simulink model "luenberg_observers"  (R2024b)
settings: Solver=VariableStepAuto  StartTime=0.0  StopTime=400  RelTol=1e-3
values from neighbouring files (symbols this model uses):
  An = double(subs(Af,{M,m1,m2,l1,l2,g},{1000,100,100,20,10,9.81}))    [PartD_LQRController.m]    (also in PartF_luenberger_observers.m; PartG_LQG_controller.m)
  Bn = double(subs(Bf,{M,m1,m2,l1,l2,g},{1000,100,100,20,10,9.81}))    [PartD_LQRController.m]    (also in PartF_luenberger_observers.m; PartG_LQG_controller.m)
  C1 = [ 0 0 0 0 0 0 ... (first row only)    [PartE_observbliltiy_check.m]    (also in PartF_luenberger_observers.m)
  C3 = [ 0 0 0 0 0 0 ... (first row only)    [PartE_observbliltiy_check.m]    (also in PartF_luenberger_observers.m)
  C4 = [ 0 0 0 0 0 0 ... (first row only)    [PartE_observbliltiy_check.m]    (also in PartF_luenberger_observers.m)
  D = [0;0;0;0;0;0]    [PartB_linearization.m]    (also in PartC_contollability_condition.m; PartD_LQRController.m; PartE_observbliltiy_check.m; PartF_luenberger_observers.m)
  x0 = [0;0;0;0;0.1;-0.1]    [PartB_linearization.m]    (also in PartC_contollability_condition.m = [0;0;0;0;0;0]; PartD_LQRController.m = [0;0;0;5;0;0]; PartE_observbliltiy_check.m = [0;0;0;0;0;0]; PartF_luenberger_observers.m = [0;0;0;0;0;0])
libraries: eeLuenbergerObserver x6

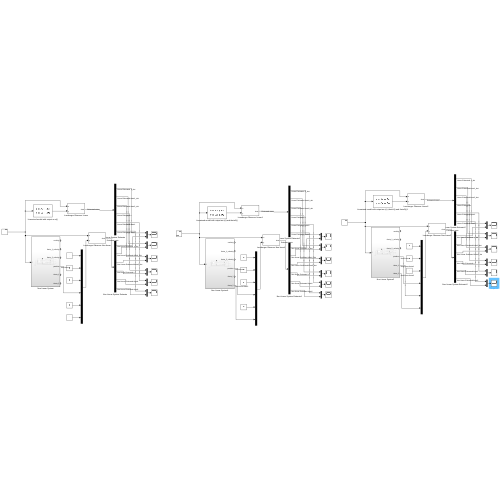
[thumbnail: Simulink's stored preview of the top-level diagram]
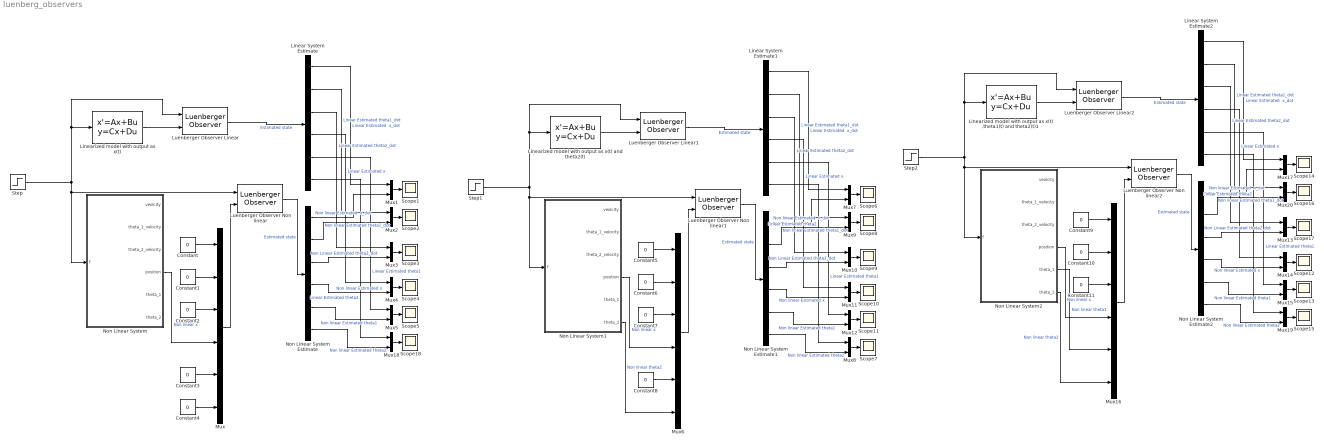
== system luenberg_observers ==
  Constant{,1..11} (12 alike) : Constant  Value=0
  Linear System Estimate : Demux  Outputs=6
  Linear System Estimate1 : Demux  Outputs=6
  Linear System Estimate2 : Demux  Outputs=6
  Linearized model with output as x(t) : StateSpace  A=An  B=Bn  C=C1  D=D  InitialCondition=x0
  Linearized model with output as x(t) ,theta1(t) and theta2(t)1 : StateSpace  A=An  B=Bn  C=C4  D=D  InitialCondition=x0
  Linearized model with output as x(t) and theta2(t) : StateSpace  A=An  B=Bn  C=C3  D=D  InitialCondition=x0
  Luenberger Observer Linear : eeLuenbergerObserver/Luenberger Observer  StateSpaceType=Continuous-time  Ad=1  Bd=1  Cd=1  Dd=1  A=An  B=Bn  C=C1  D=D  ObserverDesign=Desired eigenvalues  Ld=1  DesiredEigenvalues=poles_c1  x0=x0  Tsd=0.1  Ts=0.1
      settings: LibrarySourceBlock=ee_sl_lib/Observers/Luenberger Observer
  Luenberger Observer Linear1 : eeLuenbergerObserver/Luenberger Observer  StateSpaceType=Continuous-time  Ad=1  Bd=1  Cd=1  Dd=1  A=An  B=Bn  C=C3  D=D  ObserverDesign=Desired eigenvalues  Ld=1  DesiredEigenvalues=poles_c3  x0=x0  Tsd=0.1  Ts=0.1
      settings: LibrarySourceBlock=ee_sl_lib/Observers/Luenberger Observer
  Luenberger Observer Linear2 : eeLuenbergerObserver/Luenberger Observer  StateSpaceType=Continuous-time  Ad=1  Bd=1  Cd=1  Dd=1  A=An  B=Bn  C=C4  D=D  ObserverDesign=Desired eigenvalues  Ld=1  DesiredEigenvalues=poles_c4  x0=x0  Tsd=0.1  Ts=0.1
      settings: LibrarySourceBlock=ee_sl_lib/Observers/Luenberger Observer
  Luenberger Observer Non linear : eeLuenbergerObserver/Luenberger Observer  StateSpaceType=Continuous-time  Ad=1  Bd=1  Cd=1  Dd=1  A=An  B=Bn  C=C1  D=D  ObserverDesign=Desired eigenvalues  Ld=1  DesiredEigenvalues=poles_c1  x0=x0  Tsd=0.1  Ts=0.1
      settings: LibrarySourceBlock=ee_sl_lib/Observers/Luenberger Observer
  Luenberger Observer Non linear1 : eeLuenbergerObserver/Luenberger Observer  StateSpaceType=Continuous-time  Ad=1  Bd=1  Cd=1  Dd=1  A=An  B=Bn  C=C3  D=D  ObserverDesign=Desired eigenvalues  Ld=1  DesiredEigenvalues=poles_c3  x0=x0  Tsd=0.1  Ts=0.1
      settings: LibrarySourceBlock=ee_sl_lib/Observers/Luenberger Observer
  Luenberger Observer Non linear2 : eeLuenbergerObserver/Luenberger Observer  StateSpaceType=Continuous-time  Ad=1  Bd=1  Cd=1  Dd=1  A=An  B=Bn  C=C4  D=D  ObserverDesign=Desired eigenvalues  Ld=1  DesiredEigenvalues=poles_c4  x0=x0  Tsd=0.1  Ts=0.1
      settings: LibrarySourceBlock=ee_sl_lib/Observers/Luenberger Observer
  Mux : Mux  Inputs=6
  Mux{1..5,7..15,17..20} (18 alike) : Mux  Inputs=2
  Mux16 : Mux  Inputs=6
  Mux6 : Mux  Inputs=6
  Non Linear System : Subsystem
  Non Linear System Estimate : Demux  Outputs=6
  Non Linear System Estimate1 : Demux  Outputs=6
  Non Linear System Estimate2 : Demux  Outputs=6
  Non Linear System1 : Subsystem
  Non Linear System2 : Subsystem
  Scope{1..18} (18 alike) : Scope
  Step : Step  SampleTime=0
  Step1 : Step  SampleTime=0
  Step2 : Step  SampleTime=0
  wires:
  Step/1 -> Luenberger Observer Non linear/1, Non Linear System/1(f), Luenberger Observer Linear/1, Linearized model with output as x(t)/1
  Linearized model with output as x(t)/1 -> Luenberger Observer Linear/2
  Luenberger Observer Linear/1 -> Linear System Estimate/1  "Estimated state"
  Linear System Estimate/1 -> Mux1/1  "Linear Estimated  x_dot"
  Luenberger Observer Non linear/1 -> Non Linear System Estimate/1  "Estimated state"
  Mux/1 -> Luenberger Observer Non linear/2
  Non Linear System/4(position) -> Mux/4  "Non linear x"
  Mux1/1 -> Scope1/1
  Mux2/1 -> Scope2/1
  Mux3/1 -> Scope3/1
  Mux4/1 -> Scope4/1
  Mux5/1 -> Scope5/1
  Mux18/1 -> Scope18/1
  Linear System Estimate/2 -> Mux2/1  "Linear Estimated theta1_dot"
  Linear System Estimate/3 -> Mux3/1  "Linear Estimated theta2_dot"
  Linear System Estimate/4 -> Mux4/1  "Linear Estimated x"
  Linear System Estimate/5 -> Mux5/1  "Linear Estimated theta1"
  Linear System Estimate/6 -> Mux18/1  "Linear Estimated theta2"
  Non Linear System Estimate/1 -> Mux1/2  "Non linear Estimated  x_dot"
  Non Linear System Estimate/2 -> Mux2/2  "Non linear Estimated theta1_dot"
  Non Linear System Estimate/3 -> Mux3/2  "Non Linear Estimated theta2_dot"
  Non Linear System Estimate/4 -> Mux4/2  "Non linear Estimated x"
  Non Linear System Estimate/5 -> Mux5/2  "Non linear Estimated theta1"
  Non Linear System Estimate/6 -> Mux18/2  "Non linear Estimated theta2"
  Constant/1 -> Mux/1
  Constant1/1 -> Mux/2
  Constant2/1 -> Mux/3
  Constant3/1 -> Mux/5
  Constant4/1 -> Mux/6
  Mux12/1 -> Scope11/1
  Constant6/1 -> Mux6/2
  Non Linear System Estimate1/4 -> Mux11/2  "Non linear Estimated x"
  Mux9/1 -> Scope8/1
  Linearized model with output as x(t) and theta2(t)/1 -> Luenberger Observer Linear1/2
  Linear System Estimate1/6 -> Mux8/1  "Linear Estimated theta2"
  Constant5/1 -> Mux6/1
  Mux7/1 -> Scope6/1
  Non Linear System Estimate1/5 -> Mux12/2  "Non linear Estimated theta1"
  Non Linear System1/4(position) -> Mux6/4  "Non linear x"
  Non Linear System Estimate1/6 -> Mux8/2  "Non linear Estimated theta2"
  Non Linear System Estimate1/3 -> Mux10/2  "Non Linear Estimated theta2_dot"
  Mux11/1 -> Scope10/1
  Luenberger Observer Linear1/1 -> Linear System Estimate1/1  "Estimated state"
  Mux10/1 -> Scope9/1
  Non Linear System Estimate1/1 -> Mux7/2  "Non linear Estimated  x_dot"
  Linear System Estimate1/5 -> Mux12/1  "Linear Estimated theta1"
  Linear System Estimate1/3 -> Mux10/1  "Linear Estimated theta2_dot"
  Step1/1 -> Luenberger Observer Non linear1/1, Non Linear System1/1(f), Luenberger Observer Linear1/1, Linearized model with output as x(t) and theta2(t)/1
  Mux8/1 -> Scope7/1
  Constant8/1 -> Mux6/5
  Non Linear System Estimate1/2 -> Mux9/2  "Non linear Estimated theta1_dot"
  Linear System Estimate1/4 -> Mux11/1  "Linear Estimated x"
  Constant7/1 -> Mux6/3
  Linear System Estimate1/2 -> Mux9/1  "Linear Estimated theta1_dot"
  Mux6/1 -> Luenberger Observer Non linear1/2
  Linear System Estimate1/1 -> Mux7/1  "Linear Estimated  x_dot"
  Luenberger Observer Non linear1/1 -> Non Linear System Estimate1/1  "Estimated state"
  Non Linear System1/6(theta_2) -> Mux6/6  "Non linear theta2"
  Non Linear System Estimate2/6 -> Mux19/2  "Non linear Estimated theta2"
  Linear System Estimate2/5 -> Mux15/1  "Linear Estimated theta1"
  Constant9/1 -> Mux16/1
  Non Linear System Estimate2/3 -> Mux13/2  "Non Linear Estimated theta2_dot"
  Luenberger Observer Non linear2/1 -> Non Linear System Estimate2/1  "Estimated state"
  Mux16/1 -> Luenberger Observer Non linear2/2
  Mux15/1 -> Scope13/1
  Non Linear System Estimate2/5 -> Mux15/2  "Non linear Estimated theta1"
  Constant10/1 -> Mux16/2
  Non Linear System2/4(position) -> Mux16/4  "Non linear x"
  Non Linear System Estimate2/4 -> Mux14/2  "Non linear Estimated x"
  Linear System Estimate2/4 -> Mux14/1  "Linear Estimated x"
  Linear System Estimate2/2 -> Mux20/1  "Linear Estimated theta1_dot"
  Non Linear System Estimate2/1 -> Mux17/2  "Non linear Estimated  x_dot"
  Linearized model with output as x(t) ,theta1(t) and theta2(t)1/1 -> Luenberger Observer Linear2/2
  Non Linear System2/6(theta_2) -> Mux16/6  "Non linear theta2"
  Luenberger Observer Linear2/1 -> Linear System Estimate2/1  "Estimated state"
  Non Linear System Estimate2/2 -> Mux20/2  "Non linear Estimated theta1_dot"
  Constant11/1 -> Mux16/3
  Mux14/1 -> Scope12/1
  Mux20/1 -> Scope16/1
  Mux13/1 -> Scope17/1
  Step2/1 -> Luenberger Observer Non linear2/1, Non Linear System2/1(f), Luenberger Observer Linear2/1, Linearized model with output as x(t) ,theta1(t) and theta2(t)1/1
  Linear System Estimate2/1 -> Mux17/1  "Linear Estimated  x_dot"
  Linear System Estimate2/3 -> Mux13/1  "Linear Estimated theta2_dot"
  Mux19/1 -> Scope15/1
  Linear System Estimate2/6 -> Mux19/1  "Linear Estimated theta2"
  Mux17/1 -> Scope14/1
  Non Linear System2/5(theta_1) -> Mux16/5  "Non linear theta1"

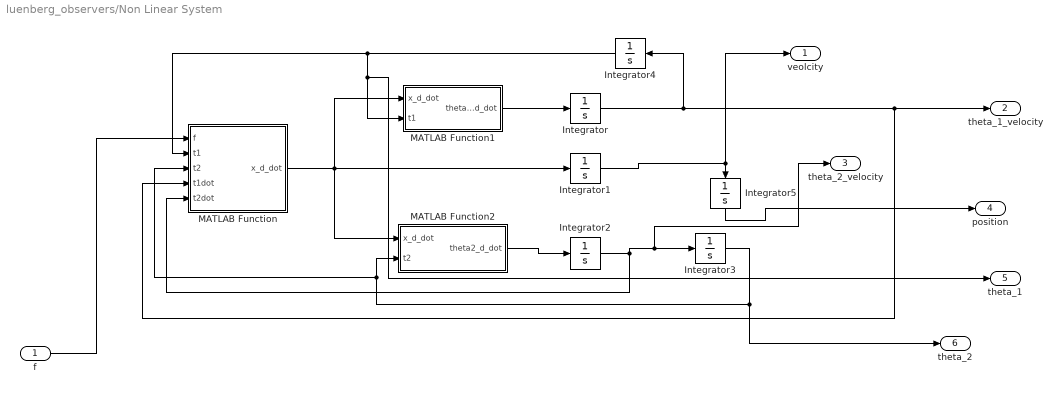
== system luenberg_observers/Non Linear System ==
  f : Inport
  Integrator : Integrator  InitialCondition=x0(2)
  Integrator1 : Integrator  InitialCondition=x0(1)
  Integrator2 : Integrator  InitialCondition=x0(3)
  Integrator3 : Integrator  InitialCondition=x0(6)
  Integrator4 : Integrator  InitialCondition=x0(5)
  Integrator5 : Integrator  InitialCondition=x0(4)
  MATLAB Function : MATLAB Function  TreatAsAtomicUnit=on
  MATLAB Function1 : MATLAB Function  TreatAsAtomicUnit=on
  MATLAB Function2 : MATLAB Function  TreatAsAtomicUnit=on
  veolcity : Outport
  theta_1_velocity : Outport  Port=2
  theta_2_velocity : Outport  Port=3
  position : Outport  Port=4
  theta_1 : Outport  Port=5
  theta_2 : Outport  Port=6
  wires:
  f/1 -> MATLAB Function/1(f)
  MATLAB Function2/1(theta2_d_dot) -> Integrator2/1
  MATLAB Function1/1(theta1_d_dot) -> Integrator/1
  Integrator5/1 -> position/1
  Integrator1/1 -> veolcity/1, Integrator5/1
  Integrator2/1 -> theta_2_velocity/1, Integrator3/1, MATLAB Function/5(t2dot)
  Integrator/1 -> Integrator4/1, theta_1_velocity/1, MATLAB Function/4(t1dot)
  Integrator4/1 -> theta_1/1, MATLAB Function1/2(t1), MATLAB Function/2(t1)
  MATLAB Function/1(x_d_dot) -> Integrator1/1, MATLAB Function1/1(x_d_dot), MATLAB Function2/1(x_d_dot)
  Integrator3/1 -> theta_2/1, MATLAB Function/3(t2), MATLAB Function2/2(t2)

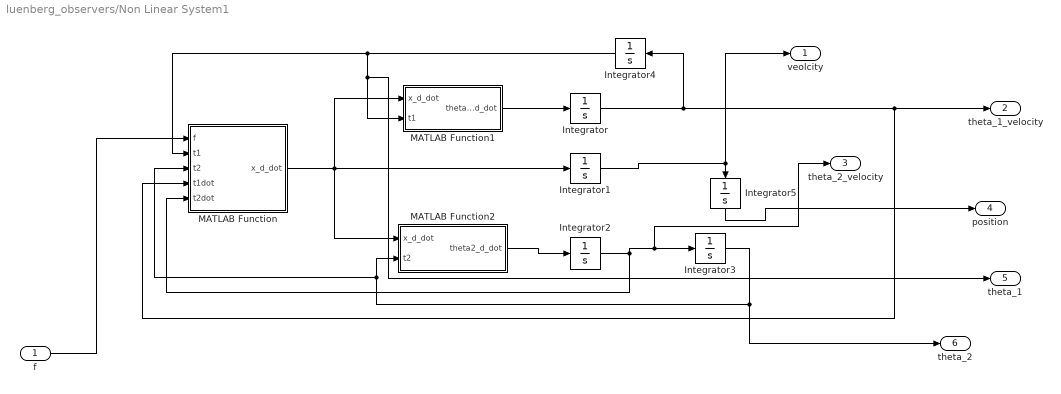
== system luenberg_observers/Non Linear System1 ==
  f : Inport
  Integrator : Integrator  InitialCondition=x0(2)
  Integrator1 : Integrator  InitialCondition=x0(1)
  Integrator2 : Integrator  InitialCondition=x0(3)
  Integrator3 : Integrator  InitialCondition=x0(6)
  Integrator4 : Integrator  InitialCondition=x0(5)
  Integrator5 : Integrator  InitialCondition=x0(4)
  MATLAB Function : MATLAB Function  TreatAsAtomicUnit=on
  MATLAB Function1 : MATLAB Function  TreatAsAtomicUnit=on
  MATLAB Function2 : MATLAB Function  TreatAsAtomicUnit=on
  veolcity : Outport
  theta_1_velocity : Outport  Port=2
  theta_2_velocity : Outport  Port=3
  position : Outport  Port=4
  theta_1 : Outport  Port=5
  theta_2 : Outport  Port=6
  wires:
  f/1 -> MATLAB Function/1(f)
  MATLAB Function2/1(theta2_d_dot) -> Integrator2/1
  MATLAB Function1/1(theta1_d_dot) -> Integrator/1
  Integrator5/1 -> position/1
  Integrator1/1 -> veolcity/1, Integrator5/1
  Integrator2/1 -> theta_2_velocity/1, Integrator3/1, MATLAB Function/5(t2dot)
  Integrator/1 -> Integrator4/1, theta_1_velocity/1, MATLAB Function/4(t1dot)
  Integrator4/1 -> theta_1/1, MATLAB Function1/2(t1), MATLAB Function/2(t1)
  MATLAB Function/1(x_d_dot) -> Integrator1/1, MATLAB Function1/1(x_d_dot), MATLAB Function2/1(x_d_dot)
  Integrator3/1 -> theta_2/1, MATLAB Function/3(t2), MATLAB Function2/2(t2)

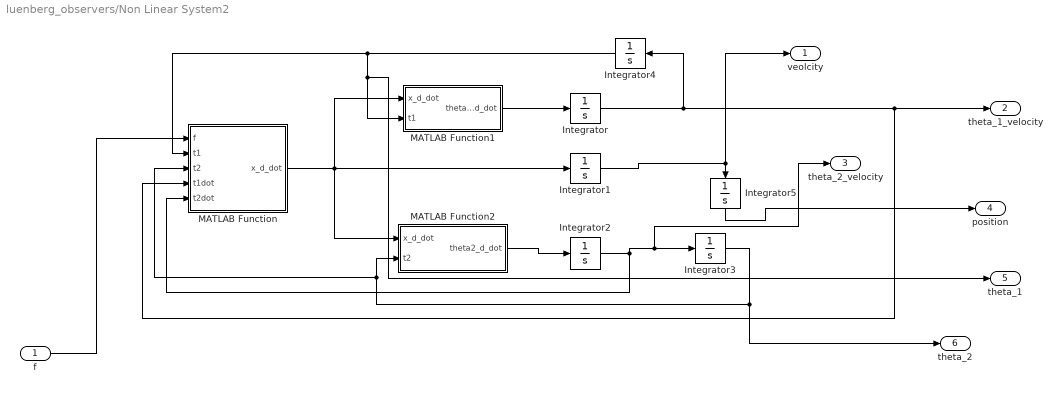
== system luenberg_observers/Non Linear System2 ==
  f : Inport
  Integrator : Integrator  InitialCondition=x0(2)
  Integrator1 : Integrator  InitialCondition=x0(1)
  Integrator2 : Integrator  InitialCondition=x0(3)
  Integrator3 : Integrator  InitialCondition=x0(6)
  Integrator4 : Integrator  InitialCondition=x0(5)
  Integrator5 : Integrator  InitialCondition=x0(4)
  MATLAB Function : MATLAB Function  TreatAsAtomicUnit=on
  MATLAB Function1 : MATLAB Function  TreatAsAtomicUnit=on
  MATLAB Function2 : MATLAB Function  TreatAsAtomicUnit=on
  veolcity : Outport
  theta_1_velocity : Outport  Port=2
  theta_2_velocity : Outport  Port=3
  position : Outport  Port=4
  theta_1 : Outport  Port=5
  theta_2 : Outport  Port=6
  wires:
  f/1 -> MATLAB Function/1(f)
  MATLAB Function2/1(theta2_d_dot) -> Integrator2/1
  MATLAB Function1/1(theta1_d_dot) -> Integrator/1
  Integrator5/1 -> position/1
  Integrator1/1 -> veolcity/1, Integrator5/1
  Integrator2/1 -> theta_2_velocity/1, Integrator3/1, MATLAB Function/5(t2dot)
  Integrator/1 -> Integrator4/1, theta_1_velocity/1, MATLAB Function/4(t1dot)
  Integrator4/1 -> theta_1/1, MATLAB Function1/2(t1), MATLAB Function/2(t1)
  MATLAB Function/1(x_d_dot) -> Integrator1/1, MATLAB Function1/1(x_d_dot), MATLAB Function2/1(x_d_dot)
  Integrator3/1 -> theta_2/1, MATLAB Function/3(t2), MATLAB Function2/2(t2)

== matlab function luenberg_observers/Non Linear System/MATLAB Function1 ==
  data: x_d_dot input; theta1_d_dot output; t1 input
function theta1_d_dot = fcn(x_d_dot,t1)

l1 = 20;
theta1_d_dot = (cos(t1)*x_d_dot - 9.81*sin(t1))/l1;

== matlab function luenberg_observers/Non Linear System/MATLAB Function ==
  data: f input; x_d_dot output; t1 input; t2 input; t1dot input; t2dot input
function x_d_dot = fcn(f,t1,t2,t1dot,t2dot)

M = 1000;
m1 = 100;
m2 = 100;
g = 9.81;
l1 = 20;
l2 = 10;

x_d_dot = (f - m1*l1*sin(t1)*t1dot^2 -m2*l2*sin(t2)*t2dot^2 -m1*g*sin(t1)*cos(t1) - m2*g*sin(t2)*cos(t2))/(M + m1*(sin(t1))^2 + m2*(sin(t2))^2);

== matlab function luenberg_observers/Non Linear System/MATLAB Function2 ==
  data: x_d_dot input; theta2_d_dot output; t2 input
function theta2_d_dot = fcn(x_d_dot,t2)

l2 = 10;
theta2_d_dot = (cos(t2)*x_d_dot - 9.81*sin(t2))/l2;

== matlab function luenberg_observers/Non Linear System1/MATLAB Function ==
  data: f input; x_d_dot output; t1 input; t2 input; t1dot input; t2dot input
function x_d_dot = fcn(f,t1,t2,t1dot,t2dot)

M = 1000;
m1 = 100;
m2 = 100;
g = 9.81;
l1 = 20;
l2 = 10;

x_d_dot = (f - m1*l1*sin(t1)*t1dot^2 -m2*l2*sin(t2)*t2dot^2 -m1*g*sin(t1)*cos(t1) - m2*g*sin(t2)*cos(t2))/(M + m1*(sin(t1))^2 + m2*(sin(t2))^2);

== matlab function luenberg_observers/Non Linear System1/MATLAB Function1 ==
  data: x_d_dot input; theta1_d_dot output; t1 input
function theta1_d_dot = fcn(x_d_dot,t1)

l1 = 20;
theta1_d_dot = (cos(t1)*x_d_dot - 9.81*sin(t1))/l1;

== matlab function luenberg_observers/Non Linear System1/MATLAB Function2 ==
  data: x_d_dot input; theta2_d_dot output; t2 input
function theta2_d_dot = fcn(x_d_dot,t2)

l2 = 10;
theta2_d_dot = (cos(t2)*x_d_dot - 9.81*sin(t2))/l2;

== matlab function luenberg_observers/Non Linear System2/MATLAB Function ==
  data: f input; x_d_dot output; t1 input; t2 input; t1dot input; t2dot input
function x_d_dot = fcn(f,t1,t2,t1dot,t2dot)

M = 1000;
m1 = 100;
m2 = 100;
g = 9.81;
l1 = 20;
l2 = 10;

x_d_dot = (f - m1*l1*sin(t1)*t1dot^2 -m2*l2*sin(t2)*t2dot^2 -m1*g*sin(t1)*cos(t1) - m2*g*sin(t2)*cos(t2))/(M + m1*(sin(t1))^2 + m2*(sin(t2))^2);

== matlab function luenberg_observers/Non Linear System2/MATLAB Function1 ==
  data: x_d_dot input; theta1_d_dot output; t1 input
function theta1_d_dot = fcn(x_d_dot,t1)

l1 = 20;
theta1_d_dot = (cos(t1)*x_d_dot - 9.81*sin(t1))/l1;

== matlab function luenberg_observers/Non Linear System2/MATLAB Function2 ==
  data: x_d_dot input; theta2_d_dot output; t2 input
function theta2_d_dot = fcn(x_d_dot,t2)

l2 = 10;
theta2_d_dot = (cos(t2)*x_d_dot - 9.81*sin(t2))/l2;
